simulink model "AllPurposeModel_TyreRelaxation"  (R2013b)
settings: Solver=ode45  StartTime=0.0  StopTime=16  FixedStep=0.001  MaxStep=0.01  RelTol=1e-3
StopFcn:
  | PlotPathAndForces(pos_irp3,delta_w4,F_z4,v_xv4,v_yv4,F_xv4,F_yv4, Par, -2);
  | TimePlots
undefined symbols (not defined in the file or in its folder): Par, sigbuilder_block
(part 2 of 2)

== matlab function AllPurposeModel_TyreRelaxation/Vehicle/Vehicle Motion/Compatibility OORP/Compatibility Eq [1.11] ==
  data: v_oorp3 input Bus: oorp_vec3; v_z4 output Bus: whl_vec4; Par parameter
function v_z4  = fcn(v_oorp3,Par)
%old: function [v_1z,v_2z,v_3z,v_4z] = fcn(v_z,w_x,w_y,Par)
%#codegen

w1=Par.Veh.TrackWidth/2;
w2=-w1;
w3=w1;
w4=w2;

lf=Par.Veh.lf;
lr=Par.Veh.lr;

v_oorp3_temp=[v_oorp3.z; v_oorp3.rotx; v_oorp3.roty];

v_oorp4=[[1;1;1;1] [w1;w2;w3;w4] [-lf;-lf;-lr;-lr]]*v_oorp3_temp;

v_z4=struct('fl',v_oorp4(1),'fr',v_oorp4(2),'rl',v_oorp4(3),'rr',v_oorp4(4));

== matlab function AllPurposeModel_TyreRelaxation/Vehicle/Wheels, Tyres & Suspsension/Tyres /Tyre Force Direction ==
  data: s_x4 input Bus: whl_vec4; s_y4 input Bus: whl_vec4; s_xy4 input; F_xyw4 input Bus: whl_vec4; F_z4_prev input Bus: whl_vec4; F_xw4 output Bus: whl_vec4; F_yw4 output Bus: whl_vec4; Par parameter
function [F_xw4,F_yw4]  = TyreModel(s_x4, s_y4, s_xy4, F_xyw4, F_z4_prev, Par)
%#codegen

F_z4_temp=[F_z4_prev.fl; F_z4_prev.fr; F_z4_prev.rl; F_z4_prev.rr];
%F_z4_temp=[Par.Veh.F_z4_static(1); Par.Veh.F_z4_static(2); Par.Veh.F_z4_static(3); Par.Veh.F_z4_static(4)];

if s_xy4.fl>Par.Env.mu/Par.Veh.C0
    F_xw4.fl=F_xyw4.fl*(+s_x4.fl/s_xy4.fl);
    F_yw4.fl=F_xyw4.fl*(-s_y4.fl/s_xy4.fl);
else
    F_xw4.fl=+F_z4_temp(1)*Par.Veh.C0*s_x4.fl; %I tried Par.Veh.F_z4_static(1) instead of F_z4.fl but too dis-continous
    F_yw4.fl=-F_z4_temp(1)*Par.Veh.C0*s_y4.fl;
end

if s_xy4.fr>Par.Env.mu/Par.Veh.C0
    F_xw4.fr=F_xyw4.fr*(+s_x4.fr/s_xy4.fr);
    F_yw4.fr=F_xyw4.fr*(-s_y4.fr/s_xy4.fr);
else
    F_xw4.fr=+F_z4_temp(2)*Par.Veh.C0*s_x4.fr;
    F_yw4.fr=-F_z4_temp(2)*Par.Veh.C0*s_y4.fr;
end

if s_xy4.rl>Par.Env.mu/Par.Veh.C0
    F_xw4.rl=F_xyw4.rl*(+s_x4.rl/s_xy4.rl);
    F_yw4.rl=F_xyw4.rl*(-s_y4.rl/s_xy4.rl);
else
    F_xw4.rl=+F_z4_temp(3)*Par.Veh.C0*s_x4.rl;
    F_yw4.rl=-F_z4_temp(3)*Par.Veh.C0*s_y4.rl;
end

if s_xy4.rr>Par.Env.mu/Par.Veh.C0
    F_xw4.rr=F_xyw4.rr*(+s_x4.rr/s_xy4.rr);
    F_yw4.rr=F_xyw4.rr*(-s_y4.rr/s_xy4.rr);
else
    F_xw4.rr=+F_z4_temp(4)*Par.Veh.C0*s_x4.rr;
    F_yw4.rr=-F_z4_temp(4)*Par.Veh.C0*s_y4.rr;
end

% if s_xy4.fl>Par.Env.mu/Par.Veh.C0
%     F_xw4.fl=F_xyw4.fl*(+s_x4.fl/s_xy4.fl);
%     F_yw4.fl=F_xyw4.fl*(-s_y4.fl/s_xy4.fl);
% else
%     F_xw4.fl=+max(F_z4.fl,0)*Par.Veh.C0*s_x4.fl;
%     F_yw4.fl=-max(F_z4.fl,0)*Par.Veh.C0*s_y4.fl;
% end
% 
% if s_xy4.fr>Par.Env.mu/Par.Veh.C0
%     F_xw4.fr=F_xyw4.fr*(+s_x4.fr/s_xy4.fr);
%     F_yw4.fr=F_xyw4.fr*(-s_y4.fr/s_xy4.fr);
% else
%     F_xw4.fr=+max(F_z4.fr,0)*Par.Veh.C0*s_x4.fr;
%     F_yw4.fr=-max(F_z4.fr,0)*Par.Veh.C0*s_y4.fr;
% end
% 
% if s_xy4.rl>Par.Env.mu/Par.Veh.C0
%     F_xw4.rl=F_xyw4.rl*(+s_x4.rl/s_xy4.rl);
%     F_yw4.rl=F_xyw4.rl*(-s_y4.rl/s_xy4.rl);
% else
%     F_xw4.rl=+max(F_z4.rl,0)*Par.Veh.C0*s_x4.rl;
%     F_yw4.rl=-max(F_z4.rl,0)*Par.Veh.C0*s_y4.rl;
% end
% 
% if s_xy4.rr>Par.Env.mu/Par.Veh.C0
%     F_xw4.rr=F_xyw4.rr*(+s_x4.rr/s_xy4.rr);
%     F_yw4.rr=F_xyw4.rr*(-s_y4.rr/s_xy4.rr);
% else
%     F_xw4.rr=+max(F_z4.rr,0)*Par.Veh.C0*s_x4.rr;
%     F_yw4.rr=-max(F_z4.rr,0)*Par.Veh.C0*s_y4.rr;
% end


% F_xw4.fl=-F_xyw4.fl*cos(atan2(s_y4.fl,-s_x4.fl));
% F_xw4.fr=-F_xyw4.fr*cos(atan2(s_y4.fr,-s_x4.fr));
% F_xw4.rl=-F_xyw4.rl*cos(atan2(s_y4.rl,-s_x4.rl));
% F_xw4.rr=-F_xyw4.rr*cos(atan2(s_y4.rr,-s_x4.rr));
% 
% F_yw4.fl=-F_xyw4.fl*sin(atan2(s_y4.fl,-s_x4.fl));
% F_yw4.fr=-F_xyw4.fr*sin(atan2(s_y4.fr,-s_x4.fr));
% F_yw4.rl=-F_xyw4.rl*sin(atan2(s_y4.rl,-s_x4.rl));
% F_yw4.rr=-F_xyw4.rr*sin(atan2(s_y4.rr,-s_x4.rr));

== matlab function AllPurposeModel_TyreRelaxation/Vehicle/Wheels, Tyres & Suspsension/Coord Transf to Vehicle/Coord Transf to veh ==
  data: F_xw4 input Bus: whl_vec4; F_yw4 input Bus: whl_vec4; F_xv4 output Bus: whl_vec4; F_yv4 output Bus: whl_vec4; delta_w4 input
function [F_xv4,F_yv4] = fcn(F_xw4, F_yw4, delta_w4)
%#codegen

F_xyv4_fl_temp=[cos(delta_w4.fl) -sin(delta_w4.fl); sin(delta_w4.fl) cos(delta_w4.fl)]*[F_xw4.fl; F_yw4.fl];
F_xyv4_fr_temp=[cos(delta_w4.fr) -sin(delta_w4.fr); sin(delta_w4.fr) cos(delta_w4.fr)]*[F_xw4.fr; F_yw4.fr];
F_xyv4_rl_temp=[cos(delta_w4.rl) -sin(delta_w4.rl); sin(delta_w4.rl) cos(delta_w4.rl)]*[F_xw4.rl; F_yw4.rl];
F_xyv4_rr_temp=[cos(delta_w4.rr) -sin(delta_w4.rr); sin(delta_w4.rr) cos(delta_w4.rr)]*[F_xw4.rr; F_yw4.rr];

F_xv4.fl=F_xyv4_fl_temp(1);
F_xv4.fr=F_xyv4_fr_temp(1);
F_xv4.rl=F_xyv4_rl_temp(1);
F_xv4.rr=F_xyv4_rr_temp(1);

F_yv4.fl=F_xyv4_fl_temp(2);
F_yv4.fr=F_xyv4_fr_temp(2);
F_yv4.rl=F_xyv4_rl_temp(2);
F_yv4.rr=F_xyv4_rr_temp(2);

== matlab function AllPurposeModel_TyreRelaxation/Vehicle/Wheels, Tyres & Suspsension/Coord Transf to Wheels /Coord Transf to whl ==
  data: v_xv4 input Bus: whl_vec4; v_xw4 output Bus: whl_vec4; v_yw4 output Bus: whl_vec4; v_yv4 input Bus: whl_vec4; delta_w4 input Bus: whl_vec4
function [v_xw4, v_yw4] = fcn(v_xv4, v_yv4, delta_w4)
%old: function [v_1xw,v_2xw,v_3xw,v_4xw, v_1yw,v_2yw,v_3yw,v_4yw] = fcn(v_1xv,v_2xv,v_3xv,v_4xv, v_1yv,v_2yv,v_3yv,v_4yv, delta_1,delta_2,delta_3,delta_4)
%#codegen

Tw1=[cos(delta_w4.fl) -sin(delta_w4.fl); sin(delta_w4.fl) cos(delta_w4.fl)];
Tw2=[cos(delta_w4.fr) -sin(delta_w4.fr); sin(delta_w4.fr) cos(delta_w4.fr)];
Tw3=[cos(delta_w4.rl) -sin(delta_w4.rl); sin(delta_w4.rl) cos(delta_w4.rl)];
Tw4=[cos(delta_w4.rr) -sin(delta_w4.rr); sin(delta_w4.rr) cos(delta_w4.rr)];

v_1xyw=Tw1'*[v_xv4.fl; v_yv4.fl];
v_2xyw=Tw2'*[v_xv4.fr; v_yv4.fr];
v_3xyw=Tw3'*[v_xv4.rl; v_yv4.rl];
v_4xyw=Tw4'*[v_xv4.rr; v_yv4.rr];

v_xw4=struct('fl',v_1xyw(1), 'fr',v_2xyw(1), 'rl',v_3xyw(1), 'rr',v_4xyw(1));
v_yw4=struct('fl',v_1xyw(2), 'fr',v_2xyw(2), 'rl',v_3xyw(2), 'rr',v_4xyw(2));

== matlab function AllPurposeModel_TyreRelaxation/Vehicle/Wheels, Tyres & Suspsension/Wheels /Wheels  ==
  data: T_s4 input Bus: whl_vec4; T_us4 input Bus: whl_vec4; derw_w4 output Bus: whl_vec4; F_xv4 input Bus: whl_vec4; F_yv4 input Bus: whl_vec4; F_z4 input Bus: whl_vec4; w_w4 input Bus: whl_vec4; Par parameter
function derw_w4 = fcn(T_s4, T_us4, F_xv4, F_yv4, F_z4, w_w4,  Par)
%old: function [derw1, derw2, derw3, derw4]  = fcn(T_1us,T_2us,T_3us,T_4us, T_1s,T_2s,T_3s,T_4s, F_1xv,F_2xv,F_3xv,F_4xv, F_1yv,F_2yv,F_3yv,F_4yv, F_z4, Par)
%#codegen

Jw=Par.Veh.Jw;

derw_w4.fl=(T_us4.fl +T_s4.fl -F_xv4.fl*Par.Veh.Rw -sign(w_w4.fl)*F_z4.fl*Par.Veh.RRC*Par.Veh.Rw)/Jw;
derw_w4.fr=(T_us4.fr +T_s4.fr -F_xv4.fr*Par.Veh.Rw -sign(w_w4.fr)*F_z4.fr*Par.Veh.RRC*Par.Veh.Rw)/Jw;
derw_w4.rl=(T_us4.rl +T_s4.rl -F_xv4.rl*Par.Veh.Rw -sign(w_w4.rl)*F_z4.rl*Par.Veh.RRC*Par.Veh.Rw)/Jw;
derw_w4.rr=(T_us4.rr +T_s4.rr -F_xv4.rr*Par.Veh.Rw -sign(w_w4.rr)*F_z4.rr*Par.Veh.RRC*Par.Veh.Rw)/Jw;

== matlab function AllPurposeModel_TyreRelaxation/Environment/Environment ==
  data: pos_irp3 input Bus: irp_vec3; Par parameter; pos_left1rel output Bus: obst_vec2; pos_left2rel output Bus: obst_vec2; pos_right1rel output Bus: obst_vec2; pos_right2rel output Bus: obst_vec2; pos_right3rel output Bus: obst_vec2
function [pos_left1rel, pos_left2rel, pos_right1rel, pos_right2rel, pos_right3rel]=Environment(pos_irp3,Par)
%#codegen

%1. obstacles (point and curves)
%1.1 relation to point obstacles, which are fixed
%1.1.1 obstacles which can be passed only one side
%1.1.1.1 obstacles on the left side of the one only possible path
pos_left1rel.x=[+cos(pos_irp3.rotz), +sin(pos_irp3.rotz)]*[Par.Env.left1.x-pos_irp3.x; Par.Env.left1.y-pos_irp3.y];
pos_left1rel.y=[-sin(pos_irp3.rotz), +cos(pos_irp3.rotz)]*[Par.Env.left1.x-pos_irp3.x; Par.Env.left1.y-pos_irp3.y];
pos_left2rel.x=[+cos(pos_irp3.rotz), +sin(pos_irp3.rotz)]*[Par.Env.left2.x-pos_irp3.x; Par.Env.left2.y-pos_irp3.y];
pos_left2rel.y=[-sin(pos_irp3.rotz), +cos(pos_irp3.rotz)]*[Par.Env.left2.x-pos_irp3.x; Par.Env.left2.y-pos_irp3.y];
%1.1.1.2 obstacles on the right side of the one only possible path
pos_right1rel.x=[+cos(pos_irp3.rotz), +sin(pos_irp3.rotz)]*[Par.Env.right1.x-pos_irp3.x; Par.Env.right1.y-pos_irp3.y];
pos_right1rel.y=[-sin(pos_irp3.rotz), +cos(pos_irp3.rotz)]*[Par.Env.right1.x-pos_irp3.x; Par.Env.right1.y-pos_irp3.y];
pos_right2rel.x=[+cos(pos_irp3.rotz), +sin(pos_irp3.rotz)]*[Par.Env.right2.x-pos_irp3.x; Par.Env.right2.y-pos_irp3.y];
pos_right2rel.y=[-sin(pos_irp3.rotz), +cos(pos_irp3.rotz)]*[Par.Env.right2.x-pos_irp3.x; Par.Env.right2.y-pos_irp3.y];
pos_right3rel.x=[+cos(pos_irp3.rotz), +sin(pos_irp3.rotz)]*[Par.Env.right3.x-pos_irp3.x; Par.Env.right3.y-pos_irp3.y];
pos_right3rel.y=[-sin(pos_irp3.rotz), +cos(pos_irp3.rotz)]*[Par.Env.right3.x-pos_irp3.x; Par.Env.right3.y-pos_irp3.y];
%1.1.2 obstacles which can be passed on either side
%NOT YET IMPLEMENTED
%Hmmm... can each of these be modelled as two with one possible passing side?

%1.2. relation to point obstacles, which are moving
%NOT YET IMPLEMENTED
%Hmmm... probably needs also relative velocity, possible acceleration

%1.3. relation to "curve obstacles" (as opposed to desired/aimed path)
%NOT YET IMPLEMENTED
%Hmmm... probably NOT good to model these as several point objects, but maybe

%2. aim points and desired path, as opposed to obstacles
%NOT YET IMPLEMENTED
%Hmmm... probably not good to implement here; should be part of driver model

== matlab function AllPurposeModel_TyreRelaxation/Vehicle/Vehicle Control & Actuators/vehicle control & actuators ==
  data: T_s4 output Bus: whl_vec4; T_us4 output Bus: whl_vec4; APed input; BPed input; SteWhlAn input; LongDir input; w_w4_actl input Bus: whl_vec4; delta_w4 output Bus: whl_vec4; Par parameter
function [T_s4, T_us4, delta_w4] = VehCtrl_Act(APed, BPed, SteWhlAn, LongDir, w_w4_actl, Par)
%#codegen

w_f_actl=(w_w4_actl.fl+w_w4_actl.fr)/2;
v_x_actl=(w_w4_actl.rl+w_w4_actl.rr)/2;

if BPed<0.01
    Fx=LongDir*APed*Par.Veh.Pmax/max([w_f_actl*Par.Veh.Rw, 1]); %LongDir is +1 or -1
elseif v_x_actl>0
    Fx=-BPed*Par.Env.mu*Par.Veh.m*Par.Env.g; %Assume prop turned off when BPed>0.01
else
    Fx=-v_x_actl*BPed*1700*9.80665; %Model as linear damping to road
end

if Fx>0
    T_s4_temp = Fx*[(Par.Veh.PropDistrFrnt/2)*[1 1] ((1-Par.Veh.PropDistrFrnt)/2)*[1 1]]*Par.Veh.Rw;
    T_us4_temp = [0 0 0 0];
else
    T_s4_temp = [0 0 0 0];
    T_us4_temp = sign(v_x_actl)*Fx*[(Par.Veh.BrkDistrFrnt/2)*[1 1] ((1-Par.Veh.BrkDistrFrnt)/2)*[1 1]]*Par.Veh.Rw;
end
delta_w4_temp = [(SteWhlAn/Par.Veh.SteRatio)*[1 1] [0 0]];

T_us4   =struct('fl',T_us4_temp(1),    'fr',T_us4_temp(2),    'rl',T_us4_temp(3),    'rr',T_us4_temp(4)   );
T_s4    =struct('fl',T_s4_temp(1),     'fr',T_s4_temp(2),     'rl',T_s4_temp(3),     'rr',T_s4_temp(4)    );
delta_w4=struct('fl',delta_w4_temp(1), 'fr',delta_w4_temp(2), 'rl',delta_w4_temp(3), 'rr',delta_w4_temp(4));
